simulink model "PLL_an_lineal"  (R2024a)
settings: Solver=VariableStepAuto  StartTime=0.0  StopTime=6  FixedStep=0.1  RelTol=1e-5  EnableMultiTasking=on
PreLoadFcn:
  | run ("Simulaciones_PLL/parametros_PLL_a.m")
InitFcn:
  | run ("Simulaciones_PLL/parametros_PLL_a.m")
values from neighbouring files (symbols this model uses):
  Cf = 1e-6    (= 1e-06)    [parametros_PLL_a.m]
  Kvco = (2*N*wi)/VDD    (= 2010.6192983)    [parametros_PLL_a.m]
  N = 32    [parametros_PLL_a.m]
  R1 = 10e3    (= 10000)    [parametros_PLL_a.m]
  R2 = 200e3    (= 200000)    [parametros_PLL_a.m]
  VDD = 10    [parametros_PLL_a.m]
settings Model: ModifiedByFormat=The MathWorks, Inc.  Creator=The MathWorks, Inc.  LastModifiedBy=The MathWorks, Inc.
settings SolverCC: MaxConsecutiveZCs=100000  ZeroCrossAlgorithm=Adaptive  AlgebraicLoopSolver=TrustRegion
settings DataIOCC: LimitDataPoints=on  MaxDataPoints=100000  SaveFormat=Array  ReturnWorkspaceOutputs=off
settings OptimizationCC: ReuseModelBlockBuffer=off  ExpressionDepthLimit=2147483647  LifeSpan=inf
settings DebuggingCC: FcnCallInpInsideContextMsg=warning  UnconnectedInputMsg=warning  UnconnectedOutputMsg=warning  UnconnectedLineMsg=warning  StateNameClashWarn=warning  SFUnexpectedBacktrackingDiag=warning  SFNoUnconditionalDefaultTransitionDiag=warning  SFExecutionAtInitializationDiag=none  ArithmeticOperatorsInVariantConditions=warning
settings HardwareCC: ProdBitPerPointer=32  ProdBitPerSizeT=32  ProdBitPerPtrDiffT=32  ProdLargestAtomicFloat=None  ProdIntDivRoundTo=Undefined  ProdEndianess=Unspecified  ProdWordSize=32  ProdHWDeviceType=32-bit Generic
settings ModelReferenceCC: EnableRefExpFcnMdlSchedulingChecks=on  PropagateSignalLabelsOutOfModel=off
settings SFSimCC: SimUseLocalCustomCode=off  CustomCodeUndefinedFunction=UseInterfaceOnly
settings RTWCC: RTWUseLocalCustomCode=off  GPUComputeCapability=3.5  DLArmComputeVersion=19.05
settings CodeAppCC: StateflowObjectComments=on
settings GRTTargetCC: TargetLangStandard=C89/C90 (ANSI)  CombineOutputUpdateFcns=off  GRTInterface=on
settings ConfigComp: CovMetricSettings=dw  CovSaveCumulativeToWorkspaceVar=on  CovSaveSingleToWorkspaceVar=on  CovExternalEMLEnable=off

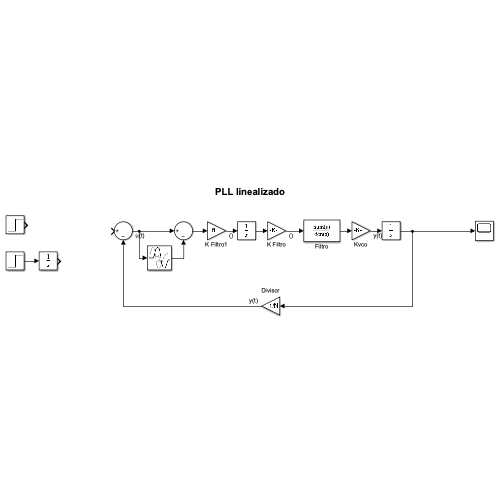
[thumbnail: Simulink's stored preview of the top-level diagram]
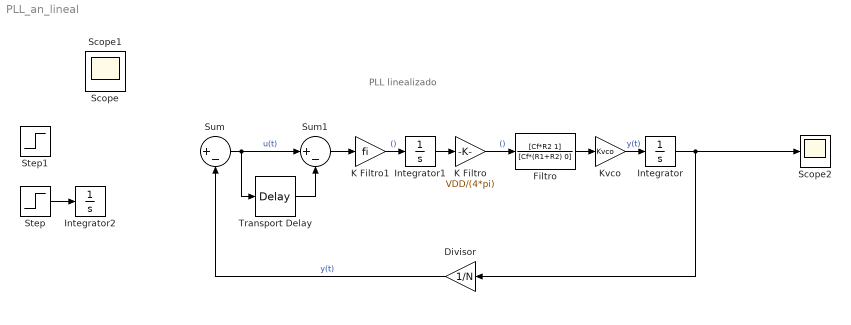
== system PLL_an_lineal ==
  note: PLL linealizado
  Divisor : Gain  Gain=1/N
  Filtro : TransferFcn  Numerator=[Cf*R2 1]  Denominator=[Cf*(R1+R2) 0]
  Integrator : Integrator
  Integrator1 : Integrator
  Integrator2 : Integrator
  K Filtro : Gain  Gain=VDD/(4*pi)
  K Filtro1 : Gain  Gain=fi
  Kvco : Gain  Gain=Kvco
  Scope2 : Scope
  Step : Step  After=pi/4  SampleTime=0
  Step1 : Step  Time=0  After=pi/2  SampleTime=0
  Sum : Sum  Inputs=|+-
  Sum1 : Sum  Inputs=|+-
  Transport Delay : TransportDelay  DelayTime=1/fi
  Scope : Scope
  Scope1 : Scope
  wires:
  Filtro/1 -> Kvco/1
  K Filtro/1 -> Filtro/1  "()"
  Kvco/1 -> Integrator/1  "y(t)"
  Integrator/1 -> Divisor/1, Scope2/1
  Sum/1 -> Transport Delay/1, Sum1/1  "u(t)"
  Transport Delay/1 -> Sum1/2
  K Filtro1/1 -> Integrator1/1  "()"
  Integrator1/1 -> K Filtro/1
  Sum1/1 -> K Filtro1/1
  Divisor/1 -> Sum/2  "y(t)"
  Step/1 -> Integrator2/1
